simulink model "p4_model"  (R2025b)
settings: Solver=VariableStepAuto  StartTime=0.0  StopTime=10.0  RelTol=1e-3
undefined symbols (not defined in the file or in its folder): carData, datBat, datCar, datMotor
libraries: autolibshared x1, slpidlib x1
(part 1 of 3)
settings Model: Creator=juanq  LastModifiedBy=KI5UXW

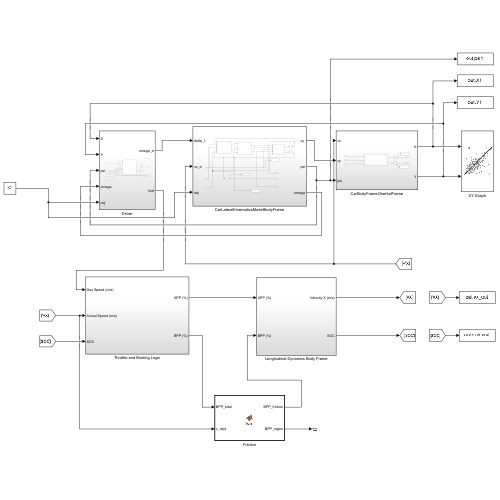
[thumbnail: Simulink's stored preview of the top-level diagram]
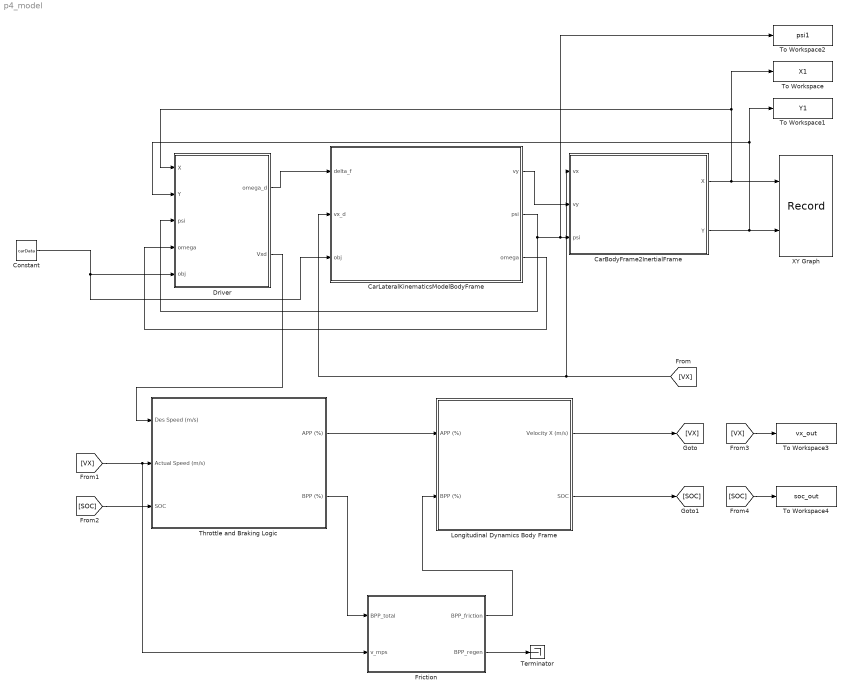
== system p4_model ==
  CarBodyFrame2InertialFrame : Subsystem
  CarLateralKinematicsModelBodyFrame : Subsystem
  Constant : Constant  Value=carData  OutDataTypeStr=Bus: slBus1
  Driver : Subsystem
  Friction : MATLAB Function  TreatAsAtomicUnit=on
  Longitudinal Dynamics Body Frame : Subsystem
  Terminator : Terminator
  "Throttle and Braking Logic " : Subsystem
  To Workspace : ToWorkspace  VariableName=X1  SaveFormat=Timeseries  SampleTime=-1
  To Workspace1 : ToWorkspace  VariableName=Y1  SaveFormat=Timeseries  SampleTime=-1
  To Workspace2 : ToWorkspace  VariableName=psi1  SaveFormat=Timeseries  SampleTime=-1
  To Workspace3 : ToWorkspace  VariableName=vx_out  SaveFormat=Timeseries  SampleTime=-1
  To Workspace4 : ToWorkspace  VariableName=soc_out  SaveFormat=Timeseries  SampleTime=-1
  XY Graph : Record  NumPorts=2.0  FileSettingsInternal="{\"entries\":[{\"content\":{\"excelSettings\":{\"content\":{},\"type\":\"Streamout.ExcelSettings\"},\"parquetSettings\":{\"content\":{},\"type\":\"Streamout.ParquetSettings\"}},\"type\":\"Streamout.FileSettingStorage\",\"uuid\":\"\"}],\"packageUris\":[\"http:\\/\\/schema.mathworks.com\\/mf0\\/streamout_blocks\\/R2020a\"],\"version\":\"1.0\"}"  FrameSettings=[0, 0]  Layout=[1 1]  SignalsInternal="{\"entries\":[{\"content\":{\"signals\":[{\"content\":{\"blockPath\":[],\"dimensions\":[1],\"domain\":\"\",\"lineColor\":\"#a2142f\",\"plots\":[ 1 ],\"port\":1,\"sid\":[\"\"],\"signalID\":1,\"signalName\":\"CarBodyFrame2InertialFrame:1\"},\"type\":\"RecordBlkView.Signal\",\"uuid\":\"\"},{\"content\":{\"blockPath\":[],\"dimensions\":[1],\"domain\":\"\",\"lineColor\":\"#139fff\",\"plots\":[ 1 ],\"port\":2,\"sid\":[\"\"],\"signalID\":2,\"signalName\":\"CarBodyFrame2InertialFrame:2\"},\"type\":\"RecordBlkView.Signal\",\"uuid\":\"\"}]},\"type\":\"RecordBlkView.InputSignals\",\"uuid\":\"\"}],\"packageUris\":[\"http:\\/\\/schema.mathworks.com\\/mf0\\/streamout_blocks\\/R2020a\"],\"version\":\"1.0\"}"  VisualizationBindings="{\"xyplotplugin\":{\"info\":[{\"series\":[{\"bindingParametersList\":[{\"parameter\":\"X-Axis\",\"signalID\":1,\"signalName\":\"CarBodyFrame2InertialFrame:1\"},{\"parameter\":\"Y-Axis\",\"signalID\":2,\"signalName\":\"CarBodyFrame2InertialFrame:2\"}],\"seriesID\":0}],\"subplotID\":1}]}}"  CompatibilityTag=XY  st=-1
  wires:
  CarBodyFrame2InertialFrame/1(X) -> XY Graph/1, To Workspace/1, Driver/1(X)
  CarLateralKinematicsModelBodyFrame/2(psi) -> Driver/3(psi), To Workspace2/1, CarBodyFrame2InertialFrame/3(psi)
  CarLateralKinematicsModelBodyFrame/3(omega) -> Driver/4(omega)
  CarBodyFrame2InertialFrame/2(Y) -> To Workspace1/1, Driver/2(Y), XY Graph/2
  Constant/1 -> CarLateralKinematicsModelBodyFrame/3(obj), Driver/5(obj)
  CarLateralKinematicsModelBodyFrame/1("vy ") -> CarBodyFrame2InertialFrame/2(vy)
  Driver/1(omega_d) -> CarLateralKinematicsModelBodyFrame/1(delta_f)
  "Throttle and Braking Logic "/2(BPP (%)) -> Friction/1(BPP_total)
  "Throttle and Braking Logic "/1(APP (%)) -> Longitudinal Dynamics Body Frame/1(APP (%))
  Longitudinal Dynamics Body Frame/1(Velocity X (m/s)) -> [VX]
  [VX] -> CarLateralKinematicsModelBodyFrame/2("vx_d "), CarBodyFrame2InertialFrame/1(vx)
  Longitudinal Dynamics Body Frame/2(SOC) -> [SOC]
  [VX] -> Friction/2(v_mps), "Throttle and Braking Logic "/2(Actual Speed (m/s))
  [SOC] -> "Throttle and Braking Logic "/3(SOC)
  Driver/2(Vxd) -> "Throttle and Braking Logic "/1("Des Speed (m/s) ")
  [VX] -> To Workspace3/1
  [SOC] -> To Workspace4/1
  Friction/1(BPP_friction) -> Longitudinal Dynamics Body Frame/2("BPP (%) ")
  Friction/2(BPP_regen) -> Terminator/1

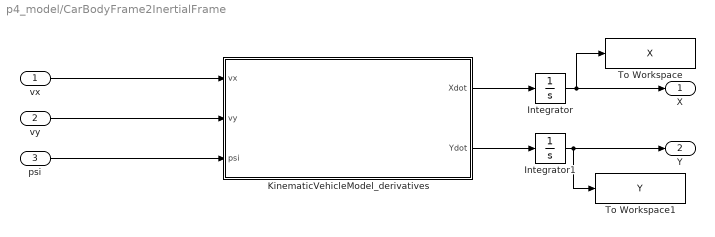
== system p4_model/CarBodyFrame2InertialFrame ==
  vx : Inport
  vy : Inport  Port=2
  psi : Inport  Port=3
  Integrator : Integrator  InitialCondition=carData.init.X0
  Integrator1 : Integrator  InitialCondition=carData.init.Y0
  KinematicVehicleModel_derivatives : MATLAB Function  TreatAsAtomicUnit=on
  To Workspace : ToWorkspace  VariableName=X  SaveFormat=Timeseries  SampleTime=-1
  To Workspace1 : ToWorkspace  VariableName=Y  SaveFormat=Timeseries  SampleTime=-1
  X : Outport
  Y : Outport  Port=2
  wires:
  KinematicVehicleModel_derivatives/1(Xdot) -> Integrator/1
  KinematicVehicleModel_derivatives/2(Ydot) -> Integrator1/1
  Integrator/1 -> To Workspace/1, X/1
  Integrator1/1 -> To Workspace1/1, Y/1
  vx/1 -> KinematicVehicleModel_derivatives/1(vx)
  vy/1 -> KinematicVehicleModel_derivatives/2(vy)
  psi/1 -> KinematicVehicleModel_derivatives/3(psi)

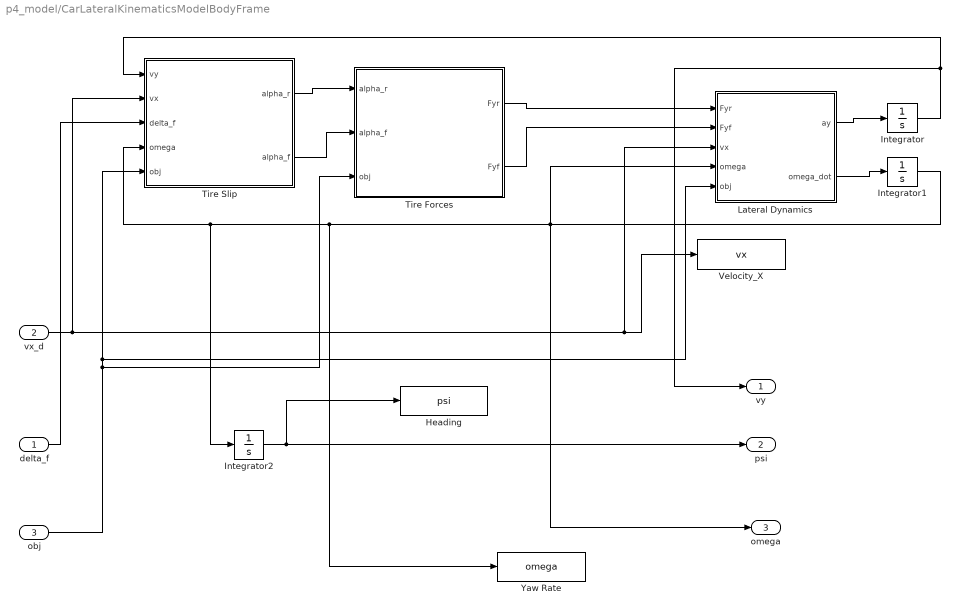
== system p4_model/CarLateralKinematicsModelBodyFrame ==
  delta_f : Inport
  "vx_d " : Inport  Port=2
  obj : Inport  Port=3
  Heading : ToWorkspace  VariableName=psi  SaveFormat=Timeseries  SampleTime=-1
  Integrator : Integrator
  Integrator1 : Integrator
  Integrator2 : Integrator
  Lateral Dynamics : MATLAB Function  TreatAsAtomicUnit=on
  Tire Forces : MATLAB Function  TreatAsAtomicUnit=on
  Tire Slip : MATLAB Function  TreatAsAtomicUnit=on
  Velocity_X : ToWorkspace  VariableName=vx  SaveFormat=Timeseries  SampleTime=-1
  Yaw Rate : ToWorkspace  VariableName=omega  SaveFormat=Timeseries  SampleTime=-1
  "vy " : Outport
  psi : Outport  Port=2
  omega : Outport  Port=3
  wires:
  Integrator2/1 -> psi/1, Heading/1
  "vx_d "/1 -> Tire Slip/2(vx), Velocity_X/1, Lateral Dynamics/3(vx)
  delta_f/1 -> Tire Slip/3(delta_f)
  Integrator/1 -> "vy "/1, Tire Slip/1(vy)
  Tire Slip/1(alpha_r) -> Tire Forces/1(alpha_r)
  Tire Slip/2(alpha_f) -> Tire Forces/2(alpha_f)
  Lateral Dynamics/1(ay) -> Integrator/1
  Lateral Dynamics/2(omega_dot) -> Integrator1/1
  Integrator1/1 -> omega/1, Lateral Dynamics/4(omega), Yaw Rate/1, Integrator2/1, Tire Slip/4(omega)
  Tire Forces/1(Fyr) -> Lateral Dynamics/1(Fyr)
  Tire Forces/2(Fyf) -> Lateral Dynamics/2(Fyf)
  obj/1 -> Tire Forces/3(obj), Lateral Dynamics/5(obj), Tire Slip/5(obj)

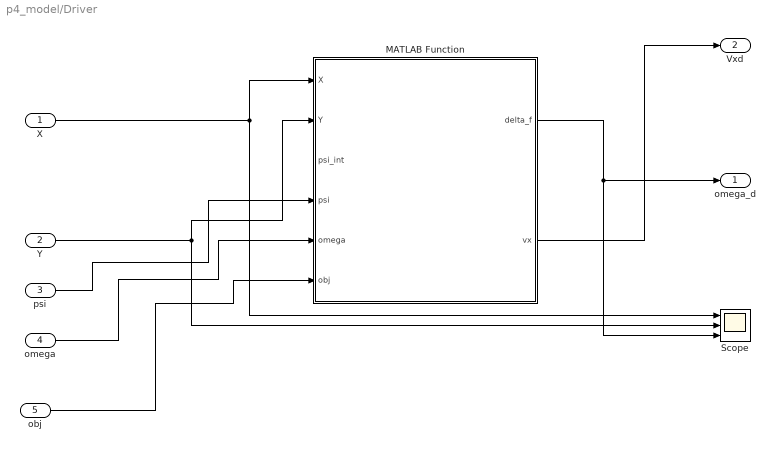
== system p4_model/Driver ==
  X : Inport
  Y : Inport  Port=2
  psi : Inport  Port=3
  omega : Inport  Port=4
  obj : Inport  Port=5
  MATLAB Function : MATLAB Function  TreatAsAtomicUnit=on
  Scope : Scope  NumInputPorts=3
      settings: ActiveDisplayYMinimum=-351.50186  ActiveDisplayYMaximum=1255.09761
  omega_d : Outport
  Vxd : Outport  Port=2
  wires:
  MATLAB Function/1(delta_f) -> omega_d/1, Scope/3
  MATLAB Function/2(vx) -> Vxd/1
  X/1 -> Scope/1, MATLAB Function/1(X)
  Y/1 -> Scope/2, MATLAB Function/2(Y)
  psi/1 -> MATLAB Function/4(psi)
  omega/1 -> MATLAB Function/5(omega)
  obj/1 -> MATLAB Function/6(obj)

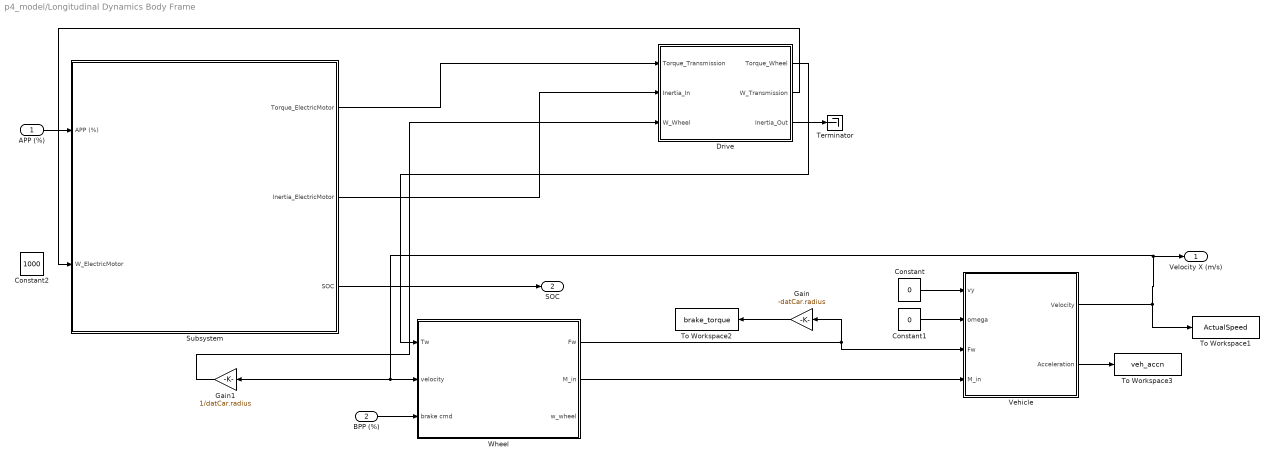
== system p4_model/Longitudinal Dynamics Body Frame ==
  APP (%) : Inport
  "BPP (%) " : Inport  Port=2
  Constant : Constant  Value=0
  Constant1 : Constant  Value=0
  Constant2 : Constant  Value=1000
  Drive : Subsystem
  Gain : Gain  Gain=-datCar.radius
  Gain1 : Gain  Gain=1/datCar.radius
  Subsystem : Subsystem
  Terminator : Terminator
  To Workspace1 : ToWorkspace  VariableName=ActualSpeed  SaveFormat=Timeseries  SampleTime=-1
  To Workspace2 : ToWorkspace  VariableName=brake_torque  SaveFormat=Timeseries  SampleTime=-1
  To Workspace3 : ToWorkspace  VariableName=veh_accn  SaveFormat=Timeseries  SampleTime=-1
  Vehicle : Subsystem
  "Wheel " : Subsystem
  Velocity X (m/s) : Outport
  SOC : Outport  Port=2
  wires:
  Vehicle/2(Acceleration) -> To Workspace3/1
  Drive/1(Torque_Wheel) -> "Wheel "/1(Tw)
  "Wheel "/2(M_in) -> Vehicle/4("M_in ")
  "BPP (%) "/1 -> "Wheel "/3(brake cmd)
  "Wheel "/1(Fw) -> Vehicle/3("Fw "), Gain/1
  Constant/1 -> Vehicle/1(vy)
  Constant1/1 -> Vehicle/2(omega)
  Vehicle/1("Velocity ") -> To Workspace1/1, Gain1/1, "Wheel "/2(velocity), Velocity X (m/s)/1
  APP (%)/1 -> Subsystem/1(APP (%))
  Subsystem/1(Torque_ElectricMotor) -> Drive/1(Torque_Transmission)
  Subsystem/2(Inertia_ElectricMotor) -> Drive/2(Inertia_In)
  Subsystem/3(SOC) -> SOC/1
  Drive/3(Inertia_Out) -> Terminator/1
  Gain/1 -> To Workspace2/1
  Drive/2(W_Transmission) -> Subsystem/2(W_ElectricMotor)
  Gain1/1 -> Drive/3(W_Wheel)

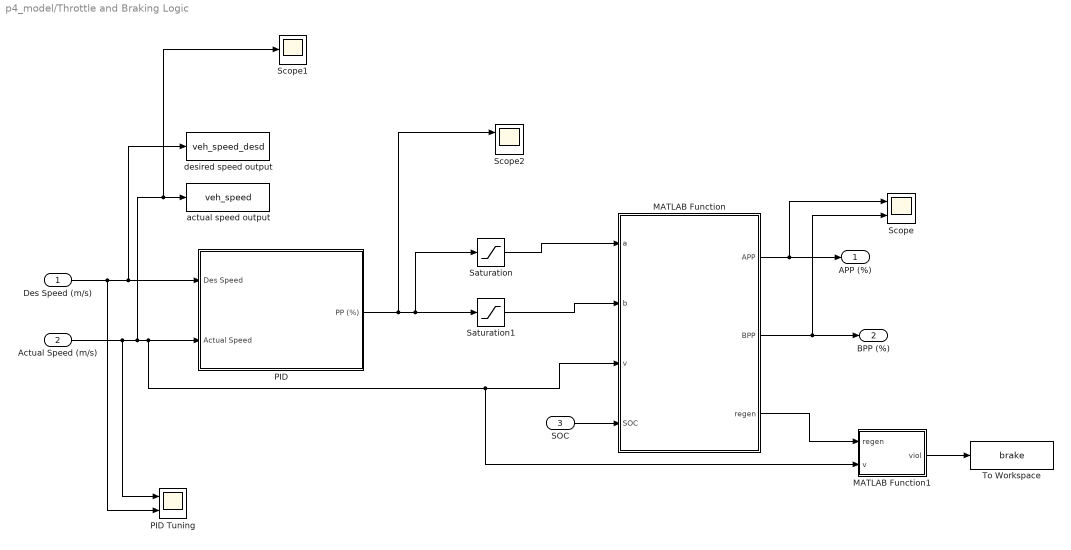
== system p4_model/Throttle and Braking Logic  ==
  "Des Speed (m/s) " : Inport
  Actual Speed (m/s) : Inport  Port=2
  SOC : Inport  Port=3
  MATLAB Function : MATLAB Function  TreatAsAtomicUnit=on
  MATLAB Function1 : MATLAB Function  TreatAsAtomicUnit=on
  PID : Subsystem
  PID Tuning : Scope  NumInputPorts=2
      settings: ActiveDisplayYMinimum=-8.2884874402324655  ActiveDisplayYMaximum=42.809426189642565
  Saturation : Saturate  UpperLimit=1  LowerLimit=0
  Saturation1 : Saturate  UpperLimit=0  LowerLimit=-1
  Scope : Scope  NumInputPorts=2
      settings: ActiveDisplayYMinimum=-0.055694331577926165  ActiveDisplayYMaximum=0.50124898420133557
  Scope1 : Scope
      settings: ActiveDisplayYMinimum=-3.08288  ActiveDisplayYMaximum=27.75461
  Scope2 : Scope  NumInputPorts=2
      settings: ActiveDisplayYMinimum=-1.0607  ActiveDisplayYMaximum=1.06103  DataLoggingVariableName=ScopeData5
  To Workspace : ToWorkspace  VariableName=brake  SaveFormat=Timeseries  SampleTime=-1
  actual speed output : ToWorkspace  VariableName=veh_speed  SaveFormat=Timeseries  SampleTime=-1
  desired speed output : ToWorkspace  VariableName=veh_speed_desd  SaveFormat=Timeseries  SampleTime=-1
  APP (%) : Outport
  BPP (%) : Outport  Port=2
  wires:
  PID/1(PP (%)) -> Scope2/1, Saturation1/1, Saturation/1
  Saturation1/1 -> MATLAB Function/2(b)
  Actual Speed (m/s)/1 -> PID Tuning/1, Scope1/1, actual speed output/1, MATLAB Function1/2(v), MATLAB Function/3(v), PID/2(Actual Speed)
  "Des Speed (m/s) "/1 -> PID Tuning/2, desired speed output/1, PID/1("Des Speed ")
  Saturation/1 -> MATLAB Function/1(a)
  MATLAB Function/1(APP) -> Scope/1, APP (%)/1
  MATLAB Function/2(BPP) -> Scope/2, BPP (%)/1
  MATLAB Function1/1(viol) -> To Workspace/1
  SOC/1 -> MATLAB Function/4(SOC)
  MATLAB Function/3(regen) -> MATLAB Function1/1(regen)

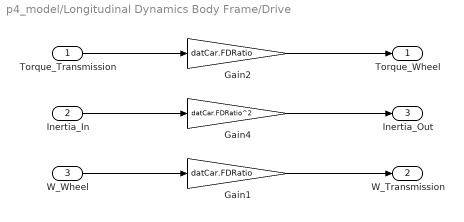
== system p4_model/Longitudinal Dynamics Body Frame/Drive ==
  Torque_Transmission : Inport
  Inertia_In : Inport  Port=2
  W_Wheel : Inport  Port=3
  Gain1 : Gain  Gain=datCar.FDRatio
  Gain2 : Gain  Gain=datCar.FDRatio
  Gain4 : Gain  Gain=datCar.FDRatio^2
  Torque_Wheel : Outport
  W_Transmission : Outport  Port=2
  Inertia_Out : Outport  Port=3
  wires:
  Torque_Transmission/1 -> Gain2/1
  Gain2/1 -> Torque_Wheel/1
  Inertia_In/1 -> Gain4/1
  Gain4/1 -> Inertia_Out/1
  W_Wheel/1 -> Gain1/1
  Gain1/1 -> W_Transmission/1

== system p4_model/Longitudinal Dynamics Body Frame/Subsystem ==
  APP (%) : Inport
  W_ElectricMotor : Inport  Port=2
  Electric Motor Drive : Subsystem
  Terminator : Terminator
  Terminator1 : Terminator
  To Workspace : ToWorkspace  VariableName=SOC  SaveFormat=Timeseries  SampleTime=-1
  Torque_ElectricMotor : Outport
  Inertia_ElectricMotor : Outport  Port=2
  SOC : Outport  Port=3
  wires:
  Electric Motor Drive/4(I_bat) -> Terminator1/1
  Electric Motor Drive/1(Torque_ElectricMotor) -> Torque_ElectricMotor/1
  Electric Motor Drive/3(V_bat) -> Terminator/1
  APP (%)/1 -> Electric Motor Drive/1(APP (%))
  Electric Motor Drive/5(SOC) -> SOC/1, To Workspace/1
  Electric Motor Drive/2(Inertia_ElectricMotor) -> Inertia_ElectricMotor/1
  W_ElectricMotor/1 -> Electric Motor Drive/2(W_ElectricMotor)

== system p4_model/Longitudinal Dynamics Body Frame/Vehicle ==
  vy : Inport
  omega : Inport  Port=2
  "Fw " : Inport  Port=3
  "M_in " : Inport  Port=4
  vehicleDragForce : Subsystem
  vehicleDynamics : Subsystem
  "Velocity " : Outport  VectorParamsAs1DForOutWhenUnconnected=off
  Acceleration : Outport  Port=2
  wires:
  vehicleDynamics/2(Out2) -> vehicleDragForce/1(vel), "Velocity "/1
  "Fw "/1 -> vehicleDynamics/1("Fw ")
  vehicleDragForce/1(Fdrag) -> vehicleDynamics/2(Fd)
  "M_in "/1 -> vehicleDynamics/3("M_in ")
  vy/1 -> vehicleDynamics/4(vy)
  omega/1 -> vehicleDynamics/5(omega)
  vehicleDynamics/1(acceleration) -> Acceleration/1
